simulink model "A1"  (R2019b)
settings: Solver=VariableStepAuto  StartTime=0.0  StopTime=15  RelTol=1e-3
libraries: simulink x4
settings Model: Creator=KK  LastModifiedBy=KK

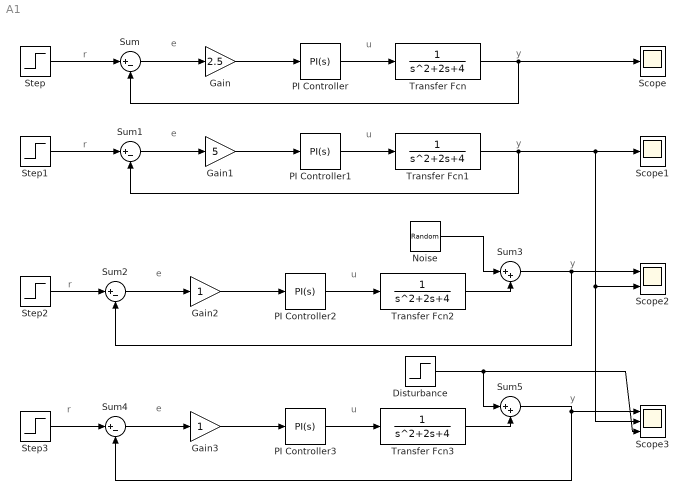
== system A1 ==
  note: y
  note: r
  note: u
  note: e
  note: y
  note: r
  note: u
  note: e
  note: y
  note: r
  note: u
  note: e
  note: y
  note: r
  note: u
  note: e
  Disturbance : Step  Time=7  After=0.15  SampleTime=0.001
  Gain : Gain  Gain=2.5
  Gain1 : Gain  Gain=5
  Gain2 : Gain
  Gain3 : Gain
  Noise : RandomNumber  Variance=0.001  Seed=34665387  SampleTime=0.001
  PI Controller{,1..3} (4 alike) : simulink/Continuous/PID Controller  Controller=PI  Form=Parallel  TimeDomain=Continuous-time  SampleTime=-1  IntegratorMethod=Forward Euler  FilterMethod=Forward Euler  ControllerParametersSource=internal  P=1  I=2  D=0  UseFilter=on  N=100  TunerSelectOption=Transfer Function Based (PID Tuner App)  InitialConditionSource=internal  InitialConditionForIntegrator=0  InitialConditionForFilter=0  DifferentiatorICPrevScaledInput=0  ExternalReset=none  TrackingMode=off  Kt=1  LimitOutput=off  UpperSaturationLimit=inf  LowerSaturationLimit=-inf  LinearizeAsGain=on  AntiWindupMode=none  Kb=1  POutMin=[]  POutMax=[]  IOutMin=[]  IOutMax=[]  DOutMin=[]  DOutMax=[]  NOutMin=[]  NOutMax=[]  SumOutMin=[]  SumOutMax=[]  SaturationOutMin=[]  SaturationOutMax=[]  PParamMin=[]  PParamMax=[]  IParamMin=[]  IParamMax=[]  DParamMin=[]  DParamMax=[]  NParamMin=[]  NParamMax=[]  KbParamMin=[]  KbParamMax=[]  KtParamMin=[]  KtParamMax=[]  KbOutMin=[]  KbOutMax=[]  KtOutMin=[]  KtOutMax=[]  IntegratorOutMin=[]  IntegratorOutMax=[]  FilterOutMin=[]  FilterOutMax=[]  SumI1OutMin=[]  SumI1OutMax=[]  SumI2OutMin=[]  SumI2OutMax=[]  SumI3OutMin=[]  SumI3OutMax=[]  SumI4OutMin=[]  SumI4OutMax=[]  SumDOutMin=[]  SumDOutMax=[]  DifferentiatorOutMin=[]  DifferentiatorOutMax=[]  FilterDiffOutCoefMin=[]  FilterDiffOutCoefMax=[]  ReciprocalOutMin=[]  ReciprocalOutMax=[]  SumDenOutMin=[]  SumDenOutMax=[]  SumNumOutMin=[]  SumNumOutMax=[]  DivideOutMin=[]  DivideOutMax=[]  IntegratorContinuousStateAttributes=''  IntegratorStateMustResolveToSignalObject=off  IntegratorRTWStateStorageClass=Auto  FilterContinuousStateAttributes=''  FilterStateMustResolveToSignalObject=off  FilterRTWStateStorageClass=Auto  ParallelPVariant=InternalParameters  IdealPVariant=Disabled  IVariant=InternalParameters  DVariant=Disabled  IntegratorVariant=Continuous  SatVariant=Disabled  AWVariant=Passthrough  PCopyVariant=Disabled  TRVariant=Disabled  FdbkBlocksVariant=Forward  IdealPFdbkVariant=Disabled  SatFdbkVariant=Disabled  DerivativeFilterVariant=Disabled  NVariant=Disabled  NCopyVariant=Disabled_SignalSpec  FilterICVariant=Disabled  IntegratorICVariant=InternalICs  ExternalResetVariant=Disabled  TRSumVariant=Passthrough  SumFdbkVariant=Disabled  SumVariant=Sum_PI
  Scope : Scope
  Scope1 : Scope
  Scope2 : Scope  NumInputPorts=2
  Scope3 : Scope  NumInputPorts=3
  Step{,1..3} (4 alike) : Step  Before=1  SampleTime=0.001
  Sum{,1..2,4} (4 alike) : Sum  Inputs=|+-
  Sum3 : Sum  Inputs=|++
  Sum5 : Sum  Inputs=|++
  Transfer Fcn{,1..3} (4 alike) : TransferFcn  Denominator=[1 2 4]
  wires:
  Gain/1 -> PI Controller/1
  Sum/1 -> Gain/1
  PI Controller/1 -> Transfer Fcn/1
  Transfer Fcn/1 -> Sum/2, Scope/1
  Step/1 -> Sum/1
  Step1/1 -> Sum1/1
  PI Controller1/1 -> Transfer Fcn1/1
  Sum1/1 -> Gain1/1
  Gain1/1 -> PI Controller1/1
  Gain2/1 -> PI Controller2/1
  Sum2/1 -> Gain2/1
  PI Controller2/1 -> Transfer Fcn2/1
  Step2/1 -> Sum2/1
  Noise/1 -> Sum3/1
  Transfer Fcn2/1 -> Sum3/2
  Sum3/1 -> Scope2/1, Sum2/2
  Sum5/1 -> Sum4/2, Scope3/1
  Transfer Fcn3/1 -> Sum5/2
  Disturbance/1 -> Sum5/1, Scope3/3
  Step3/1 -> Sum4/1
  PI Controller3/1 -> Transfer Fcn3/1
  Sum4/1 -> Gain3/1
  Gain3/1 -> PI Controller3/1
  Transfer Fcn1/1 -> Scope2/2, Scope3/2, Scope1/1, Sum1/2
